simulink model "linear_balan_bot_disc"  (R2018b)
settings: Solver=FixedStepDiscrete  StartTime=0.0  StopTime=10.0  FixedStep=0.001  RelTol=1e-3
undefined symbols (not defined in the file or in its folder): d_P_cart_den, d_P_cart_num, d_P_pend_den, d_P_pend_num
libraries: simulink_extras x2, simulink x1
settings Model: Creator=Ikarus  LastModifiedBy=Ikarus

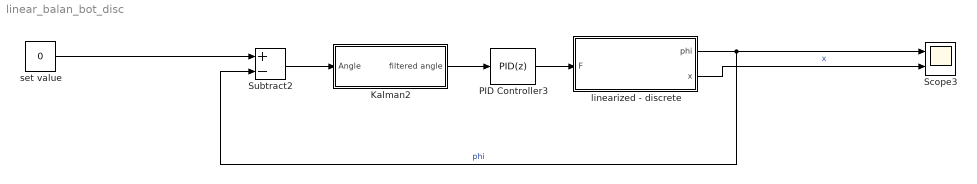
== system linear_balan_bot_disc ==
  Kalman2 : Subsystem  mask{step_time=0.01}
      mask prompts: step_time "step time"
  PID Controller3 : simulink/Continuous/PID Controller  Controller=PID  Form=Parallel  TimeDomain=Discrete-time  SampleTime=-1  IntegratorMethod=Forward Euler  FilterMethod=Forward Euler  ControllerParametersSource=internal  P=789.794814229085  I=503.452349337569  D=303.317596444162  UseFilter=on  N=74.1133672012099  TunerSelectOption=Transfer Function Based (PID Tuner App)  InitialConditionSource=internal  InitialConditionForIntegrator=0  InitialConditionForFilter=0  DifferentiatorICPrevScaledInput=0  ExternalReset=none  TrackingMode=off  Kt=1  LimitOutput=off  UpperSaturationLimit=inf  LowerSaturationLimit=-inf  LinearizeAsGain=on  AntiWindupMode=none  Kb=1  POutMin=[]  POutMax=[]  IOutMin=[]  IOutMax=[]  DOutMin=[]  DOutMax=[]  NOutMin=[]  NOutMax=[]  SumOutMin=[]  SumOutMax=[]  SaturationOutMin=[]  SaturationOutMax=[]  PParamMin=[]  PParamMax=[]  IParamMin=[]  IParamMax=[]  DParamMin=[]  DParamMax=[]  NParamMin=[]  NParamMax=[]  KbParamMin=[]  KbParamMax=[]  KtParamMin=[]  KtParamMax=[]  KbOutMin=[]  KbOutMax=[]  KtOutMin=[]  KtOutMax=[]  IntegratorOutMin=[]  IntegratorOutMax=[]  FilterOutMin=[]  FilterOutMax=[]  SumI1OutMin=[]  SumI1OutMax=[]  SumI2OutMin=[]  SumI2OutMax=[]  SumI3OutMin=[]  SumI3OutMax=[]  SumI4OutMin=[]  SumI4OutMax=[]  SumDOutMin=[]  SumDOutMax=[]  DifferentiatorOutMin=[]  DifferentiatorOutMax=[]  FilterDiffOutCoefMin=[]  FilterDiffOutCoefMax=[]  ReciprocalOutMin=[]  ReciprocalOutMax=[]  SumDenOutMin=[]  SumDenOutMax=[]  SumNumOutMin=[]  SumNumOutMax=[]  DivideOutMin=[]  DivideOutMax=[]  IntegratorContinuousStateAttributes=''  IntegratorStateMustResolveToSignalObject=off  IntegratorRTWStateStorageClass=Auto  FilterContinuousStateAttributes=''  FilterStateMustResolveToSignalObject=off  FilterRTWStateStorageClass=Auto  ParallelPVariant=InternalParameters  IdealPVariant=Disabled  IVariant=InternalParameters  DVariant=InternalParameters  IntegratorVariant=Discrete  SatVariant=Disabled  AWVariant=Passthrough  PCopyVariant=Disabled  TRVariant=Disabled  FdbkBlocksVariant=Forward  IdealPFdbkVariant=Disabled  SatFdbkVariant=Disabled  DerivativeFilterVariant=ForwardEulerFilter  NVariant=InternalParameters  NCopyVariant=Disabled  FilterICVariant=InternalICsFilter  IntegratorICVariant=InternalICs  ExternalResetVariant=Disabled  TRSumVariant=Passthrough  SumFdbkVariant=Disabled  SumVariant=Sum_PID
  Scope3 : Scope  NumInputPorts=2
  Subtract2 : Sum  Inputs=+-
  linearized - discrete : Subsystem
  set value : Constant  Value=0  SampleTime=-1
  wires:
  set value/1 -> Subtract2/1
  Subtract2/1 -> Kalman2/1("Angle ")
  linearized - discrete/1(phi) -> Subtract2/2, Scope3/1  "phi"
  Kalman2/1(filtered angle) -> PID Controller3/1
  PID Controller3/1 -> linearized - discrete/1(F)
  linearized - discrete/2(x) -> Scope3/2  "x"

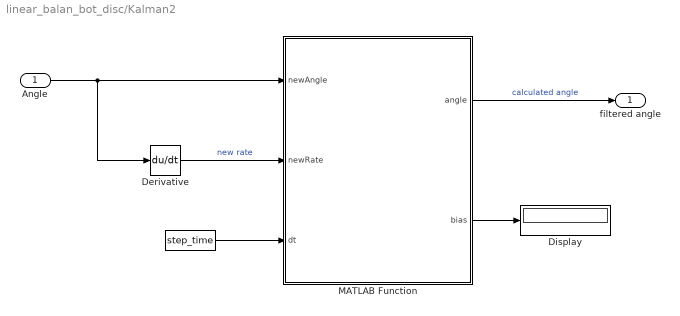
== system linear_balan_bot_disc/Kalman2 ==
  "Angle " : Inport
  "  " : Constant  Value=step_time  SampleTime=-1
  Derivative : Derivative  CoefficientInTFapproximation=-1
  Display : Display
  MATLAB Function : MATLAB Function  TreatAsAtomicUnit=on
  filtered angle : Outport
  wires:
  MATLAB Function/2(bias) -> Display/1
  "Angle "/1 -> MATLAB Function/1(newAngle), Derivative/1
  MATLAB Function/1(angle) -> filtered angle/1  "calculated angle"
  Derivative/1 -> MATLAB Function/2(newRate)  "new rate"
  "  "/1 -> MATLAB Function/3(dt)

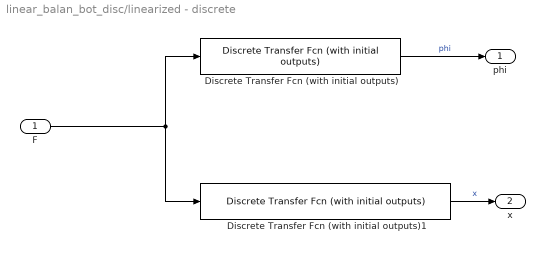
== system linear_balan_bot_disc/linearized - discrete ==
  F : Inport
  Discrete Transfer Fcn (with initial outputs) : simulink_extras/Additional Discrete/Discrete Transfer Fcn (with initial outputs)  N=[d_P_pend_num]  D=[d_P_pend_den]  U0=0  Y0=10*pi/180  TS=-1
      settings: SourceProductName=Simulink  SourceProductBaseCode=SL
  Discrete Transfer Fcn (with initial outputs)1 : simulink_extras/Additional Discrete/Discrete Transfer Fcn (with initial outputs)  N=[d_P_cart_num]  D=[d_P_cart_den]  U0=0  Y0=0  TS=-1
      settings: SourceProductName=Simulink  SourceProductBaseCode=SL
  phi : Outport
  x : Outport  Port=2
  wires:
  F/1 -> Discrete Transfer Fcn (with initial outputs)/1, Discrete Transfer Fcn (with initial outputs)1/1
  Discrete Transfer Fcn (with initial outputs)1/1 -> x/1  "x"
  Discrete Transfer Fcn (with initial outputs)/1 -> phi/1  "phi"

== matlab function linear_balan_bot_disc/Kalman2/MATLAB Function ==
  settings: updateMethod=DISCRETE
  data: newAngle input; angle output; newRate input; dt input; bias output
function [angle,bias] = KalmanFil_Balanbot(newAngle,newRate,dt)
        % This script was adapted for its implementation in Simulink by R. Estrada (FH JOANNEUM 2017)
        % Based on KasBot V2  -  Kalman filter module - http:%www.x-firm.com/?page_id=145
        % Modified by Kristian Lauszus
        % More information: http:%blog.tkjelectronics.dk/2012/09/a-practical-approach-to-kalman-filter-and-how-to-implement-it

        % Discrete Kalman filter time update equations - Time Update ("Predict")
        % Update xhat - Project the state ahead
        
        coder.extrinsic('exist');
        
        % Declaration of persistent in memory variables (similar to declare global
        % variables)
   
        persistent init0 P K x;        
        
        % Initialization of typical sensor and noise variances 
        Q_angle = 0.001;
        Q_bias = 0.003; 
        R_measure = 0.03;
        
        % Declaration/initialization of main static matrices and vectors
        F = [1      -dt; 0      1];     % Transition matrix
        Q = [Q_angle  0; 0 Q_bias];     % Process noise covariance matrix  
        B = [dt ; 0];                   % Control-input model
        H = [1    0];                   % Observation model
        
        % SETUP: Executed only the first time      
        if isempty(init0)
            init0=0;
             % Declaration/initialization of main dynamic matrix and vectors
            P     = [0 0;0 0];  % Error covariance matrix
            K     = [0;0];      % Kalman gain vector
            x     = [0;0];      % State vector
        end

        % LOOP: Implementation of Kalman filter algorithm
        
        % Step 1 */          
        % Calculate prior state vector
        x = F * x + B * newRate;        

        % Step 2 */ 
        % Update estimation error covariance - Project the error covariance ahead               
         P = F * P * F' + Q * dt;  
                   
        % Step 3 */
        % Update estimate with measurement zk (newAngle)     
        y = newAngle - H * x;
        
        % Step 4 */
        % Discrete Kalman filter measurement update equations - Measurement Update ("Correct")              
        S = H * P * H' + R_measure;
        
        % Step 5 */
        % Compute the Kalman gain  
        K = P * H' / S;

        % Step 6 */
        % Update state vector
        x = x + K * y;
        
        % Step 7 */
        % Calculate estimation error covariance - Update the error covariance
        P = (eye(2) - K * H) * P;

        % RETURN: Update the function outputs
        angle = x(1);
        bias  = x(2);
